simulink model "train"  (R2023b)
settings: Solver=ode45  StartTime=0.0  StopTime=1000  RelTol=1e-3
values from neighbouring files (symbols this model uses):
  g = 9.81    [test1.m]
  k = 1    [test1.m]
  M1 = 1    [test1.m]
  M2 = 0.5    [test1.m]
settings Model: Creator=sansh  LastModifiedBy=musta
settings SolverCC: AlgebraicLoopSolver=TrustRegion
settings DataIOCC: ReturnWorkspaceOutputs=off
settings DebuggingCC: UnconnectedInputMsg=warning  UnconnectedOutputMsg=warning  UnconnectedLineMsg=warning  ArithmeticOperatorsInVariantConditions=warning
settings ModelReferenceCC: EnableRefExpFcnMdlSchedulingChecks=on
settings SFSimCC: SimUseLocalCustomCode=off  CustomCodeUndefinedFunction=UseInterfaceOnly
settings RTWCC: RTWUseLocalCustomCode=off
settings CodeAppCC: StateflowObjectComments=on

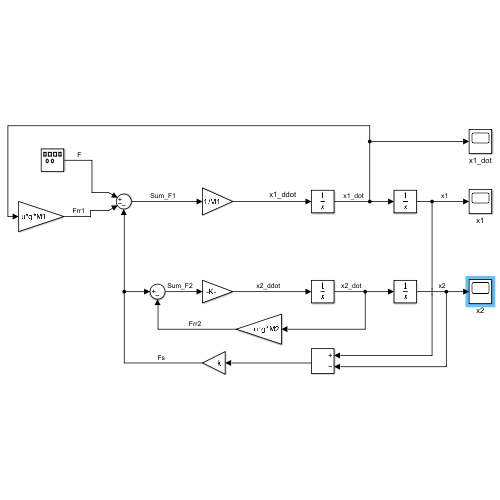
[thumbnail: Simulink's stored preview of the top-level diagram]
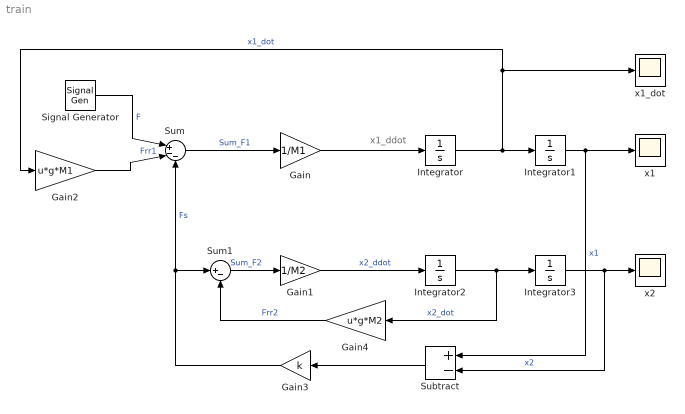
== system train ==
  note: x1_ddot
  Gain : Gain  Gain=1/M1
  Gain1 : Gain  Gain=1/M2
  Gain2 : Gain  Gain=u*g*M1
  Gain3 : Gain  Gain=k
  Gain4 : Gain  Gain=u*g*M2
  Integrator{,1..3} (4 alike) : Integrator
  Signal Generator : SignalGenerator  WaveForm=square  Amplitude=-1  Frequency=0.001
  Subtract : Sum  Inputs=+-
  Sum : Sum  Inputs=|+--
  Sum1 : Sum  Inputs=|+-
  x1 : Scope
  x1_dot : Scope
  x2 : Scope
  wires:
  Sum/1 -> Gain/1  "Sum_F1"
  Sum1/1 -> Gain1/1  "Sum_F2"
  Gain/1 -> Integrator/1
  Integrator/1 -> x1_dot/1, Gain2/1, Integrator1/1  "x1_dot"
  Gain1/1 -> Integrator2/1  "x2_ddot"
  Integrator2/1 -> Gain4/1, Integrator3/1  "x2_dot"
  Integrator1/1 -> Subtract/1, x1/1  "x1"
  Integrator3/1 -> Subtract/2, x2/1  "x2"
  Signal Generator/1 -> Sum/1  "F"
  Gain2/1 -> Sum/2  "Frr1"
  Subtract/1 -> Gain3/1
  Gain3/1 -> Sum1/1, Sum/3  "Fs"
  Gain4/1 -> Sum1/2  "Frr2"
